simulink model "board_specific_NUCLEO_F446_SPISlave_Master"  (R2016b)
settings: Solver=FixedStepDiscrete  StartTime=0.0  StopTime=10.0  FixedStep=1e-3  RelTol=1e-3
libraries: mbed_lib x5, simulink x2
settings Model: Creator=oh  LastModifiedBy=oh
settings OptimizationCC: DefaultParameterBehavior=Inlined
settings DebuggingCC: ParameterTunabilityLossMsg=error
settings HardwareCC: ProdBitPerPointer=32  ProdBitPerSizeT=32  ProdBitPerPtrDiffT=32  ProdLargestAtomicInteger=Long  ProdLargestAtomicFloat=Double  ProdWordSize=32  ProdHWDeviceType=ARM Compatible->ARM Cortex
settings RTWCC: SystemTargetFile=mbed.tlc  TemplateMakefile=mbed.tmf  Description=Mbed Target (Embedded Target)  GenerateReport=on  IncludeHyperlinkInReport=on  LaunchReport=on  TargetLang=C++  GenerateTraceInfo=on  GenerateTraceReport=on  GenerateTraceReportSl=on  GenerateTraceReportSf=on  GenerateTraceReportEml=on
settings CodeAppCC: ForceParamTrailComments=on  IgnoreCustomStorageClasses=off  OperatorAnnotations=on  SimulinkDataObjDesc=on  SFDataObjDesc=on  MATLABFcnDesc=on  InsertBlockDesc=on  MATLABSourceComments=on
settings STFCustomTargetCC: TargetLibSuffix=.a  TargetLangStandard=C++03 (ISO)  GenerateSampleERTMain=on  CombineOutputUpdateFcns=on  ERTCustomFileBanners=on  SupportContinuousTime=off  SupportNonInlinedSFcns=off  RemoveResetFunc=on  MATLABClassNameForMDSCustomization=Simulink.SoftwareTarget.ERTCustomization  GRTInterface=off  SystemTargetFile=mbed.tlc
settings ERTTargetCC: TargetLangStandard=C++03 (ISO)  GenerateSampleERTMain=on  ParMdlRefBuildCompliant=off  CompOptLevelCompliant=off  ConcurrentExecutionCompliant=off  ERTFirstTimeCompliant=off  ModelStepFunctionPrototypeControlCompliant=off  CPPClassGenCompliant=off  UseToolchainInfoCompliant=off  InlinedParameterPlacement=NonHierarchical  ERTCustomFileTemplate=mbed_file_process.tlc

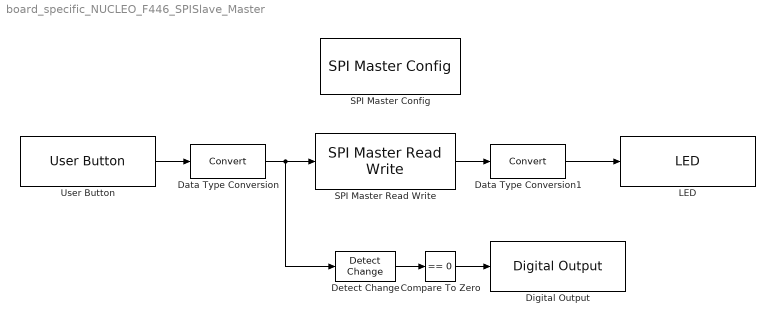
== system board_specific_NUCLEO_F446_SPISlave_Master ==
  Compare To Zero : simulink/Logic and Bit Operations/Compare To Zero  relop===  OutDataTypeStr=uint8
  Data Type Conversion : DataTypeConversion
  Data Type Conversion1 : DataTypeConversion
  Detect Change : simulink/Logic and Bit Operations/Detect Change  vinit=0  OutDataTypeStr=boolean
  Digital Output : mbed_lib/GPIO/Digital Output  PortName=A  PinNumber=0  OutputMode=PullDefault  SampleTime=-1
  LED : mbed_lib/GPIO/LED  nLED=1  SampleTime=-1
  SPI Master Config : mbed_lib/Serial/SPI/SPI Master Config  Priority=0  SPIPort=1  Freq=100000  Mode=0  Bits=8  MOSIPortNameShow=NC  MOSIPortName=-1  MOSIPinNumber=7  MISOPortNameShow=A  MISOPortName=0  MISOPinNumber=6  SCLKPortName=A  Parameter13=0  SCLKPinNumber=5
  SPI Master Read Write : mbed_lib/Serial/SPI/SPI Master Read Write  SpiPort=1  CsPort=B  CsPin=6
  User Button : mbed_lib/GPIO/User Button  SampleTime=-1
  wires:
  User Button/1 -> Data Type Conversion/1
  SPI Master Read Write/1 -> Data Type Conversion1/1
  Compare To Zero/1 -> Digital Output/1
  Detect Change/1 -> Compare To Zero/1
  Data Type Conversion/1 -> SPI Master Read Write/1, Detect Change/1
  Data Type Conversion1/1 -> LED/1
